simulink model "robot_step_8"  (R2020b)
settings: Solver=VariableStepAuto  StartTime=0.0  StopTime=2  RelTol=1e-3
libraries: roblocks x3

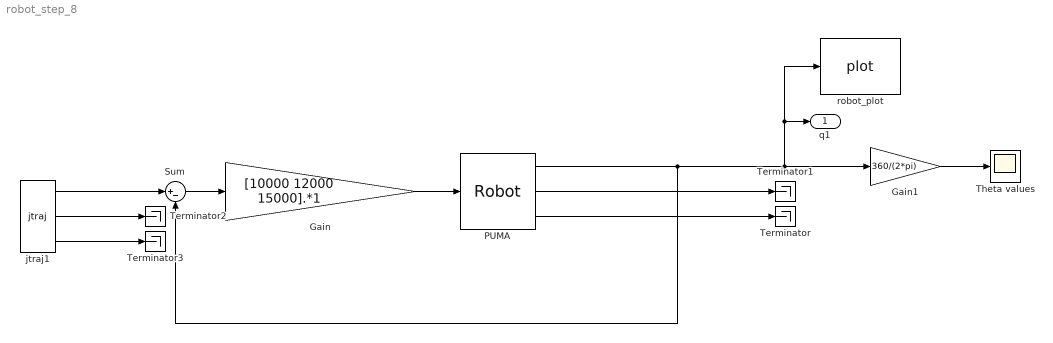
== system robot_step_8 ==
  Gain : Gain  Gain=[10000 12000 15000].*1
  Gain1 : Gain  Gain=360/(2*pi)
  PUMA : roblocks/Arm/Robot  robot=robot  q0=[0 0 0]
  Sum : Sum  Inputs=|+-
  Terminator{,1..3} (4 alike) : Terminator
  Theta values : Scope
  jtraj1 : roblocks/Toolbox/jtraj  q0=[0 0 0]  qf=[pi/2 -pi/4 -pi/4]  tmax=2  ts=0.02
  robot_plot : roblocks/Arm/plot  robot=robot  fps=5  holdplot=on
  q1 : Outport
  wires:
  PUMA/1 -> Sum/2, robot_plot/1, q1/1, Gain1/1
  Gain/1 -> PUMA/1
  Gain1/1 -> Theta values/1
  Sum/1 -> Gain/1
  jtraj1/1 -> Sum/1
  PUMA/3 -> Terminator/1
  PUMA/2 -> Terminator1/1
  jtraj1/2 -> Terminator2/1
  jtraj1/3 -> Terminator3/1
